simulink model "task3"  (R2024a)
settings: Solver=VariableStepAuto  StartTime=0.0  StopTime=10  RelTol=1e-3
libraries: cstblocks x3
settings Model: Creator=lalayants  LastModifiedBy=lalayants

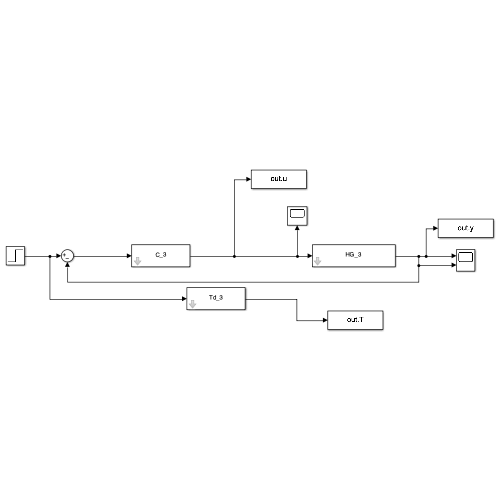
[thumbnail: Simulink's stored preview of the top-level diagram]
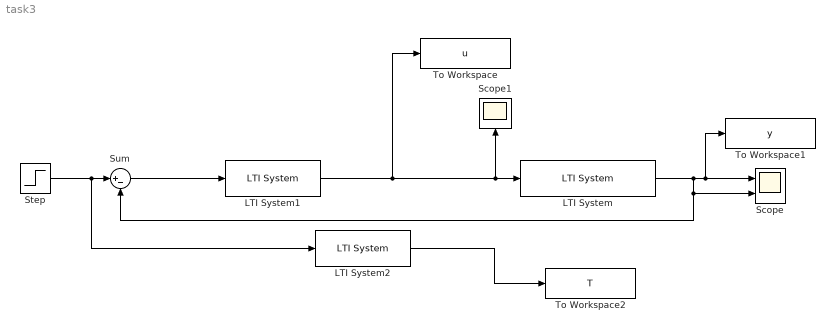
== system task3 ==
  LTI System : cstblocks/LTI System  sys=HG_3  IC=[]  PadeOrder=0
  LTI System1 : cstblocks/LTI System  sys=C_3  IC=[]  PadeOrder=0
  LTI System2 : cstblocks/LTI System  sys=Td_3  IC=[]  PadeOrder=0
  Scope : Scope  NumInputPorts=2
  Scope1 : Scope
  Step : Step  Time=0  SampleTime=0
  Sum : Sum  Inputs=|+-
  To Workspace : ToWorkspace  VariableName=u  SaveFormat=Timeseries  SampleTime=-1
  To Workspace1 : ToWorkspace  VariableName=y  SaveFormat=Timeseries  SampleTime=-1
  To Workspace2 : ToWorkspace  VariableName=T  SaveFormat=Timeseries  SampleTime=-1
  wires:
  Step/1 -> LTI System2/1, Sum/1
  Sum/1 -> LTI System1/1
  LTI System/1 -> To Workspace1/1, Scope/1, Sum/2, Scope/2
  LTI System1/1 -> To Workspace/1, LTI System/1, Scope1/1
  LTI System2/1 -> To Workspace2/1
